simulink model "c"  (R2023a)
settings: Solver=ode4  StartTime=0.0  StopTime=15  FixedStep=0.002  RelTol=1e-3
InitFcn:
  | init;
undefined symbols (not defined in the file): g, N, T, v_c
libraries: dspsrcs4 x2
settings Model: Creator=Ali  LastModifiedBy=Ali

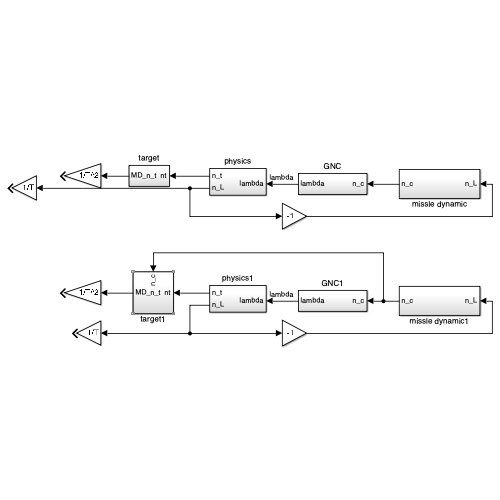
[thumbnail: Simulink's stored preview of the top-level diagram]
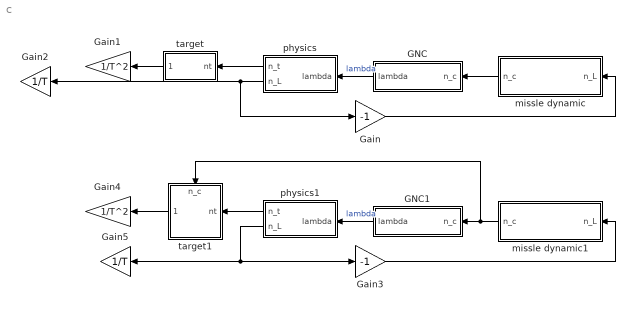
== system c ==
  GNC : Subsystem
  GNC1 : Subsystem
  Gain : Gain  Gain=-1
  Gain1 : Gain  Gain=1/T^2
  Gain2 : Gain  Gain=1/T
  Gain3 : Gain  Gain=-1
  Gain4 : Gain  Gain=1/T^2
  Gain5 : Gain  Gain=1/T
  missle dynamic : Subsystem
  missle dynamic1 : Subsystem
  physics : Subsystem
  physics1 : Subsystem
  target : Subsystem
  target1 : Subsystem
      settings: PortSchema="{\"entries\":[{\"content\":{\"sides\":[{\"content\":{\"connectorIds\":[\"In1\"]},\"type\":\"ConnectorPlacement.EquallySpacedRectSide\",\"uuid\":\"ed75f11e-c865-4004-9925-7377fa04d387\"},{\"content\":{\"connectorIds\":[\"Out1\"],\"side\":\"RIGHT\"},\"type\":\"ConnectorPlacement.EquallySpacedRectSide\",\"uuid\":\"bae2f0f6-1e21-4a13-88c5-2ae7c6156ea9\"},{\"content\":{\"connectorIds\":[\"In2\"],\"side\":\"TOP\"},\"type\":\"ConnectorPlacement.EquallySpacedRectSide\",\"uuid\":\"941d1b82-2a2d-4b33-9910-844af34ed272\"}]},\"type\":\"ConnectorPlacement.EquallySpacedConnector\",\"uuid\":\"c15f6690-1bd4-4323-98c9-9e5b3f44ccd0\"}],\"packageUris\":[\"http://schema.mathworks.com/mf0/Connector/R2020b\"],\"version\":\"1.0\"}"
  wires:
  GNC/1(lambda) -> physics/1(lambda)  "lambda"
  physics/2(n_L) -> Gain2/1, Gain/1
  missle dynamic/1(n_c) -> GNC/1(n_c)
  target/1(MD_n_t) -> Gain1/1
  physics/1(n_t) -> target/1(nt)
  Gain/1 -> missle dynamic/1(n_L)
  target1/1(MD_n_t) -> Gain4/1
  GNC1/1(lambda) -> physics1/1(lambda)  "lambda"
  physics1/1(n_t) -> target1/1(nt)
  physics1/2(n_L) -> Gain5/1, Gain3/1
  missle dynamic1/1(n_c) -> target1/2(n_c), GNC1/1(n_c)
  Gain3/1 -> missle dynamic1/1(n_L)

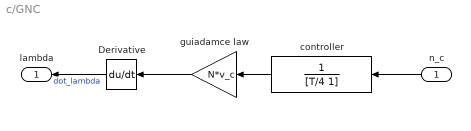
== system c/GNC ==
  n_c : Inport
  Derivative : Derivative
  controller : TransferFcn  Denominator=[T/4 1]
  guiadamce law : Gain  Gain=N*v_c
  lambda : Outport
  wires:
  Derivative/1 -> lambda/1  "dot_lambda"
  n_c/1 -> controller/1
  controller/1 -> guiadamce law/1
  guiadamce law/1 -> Derivative/1

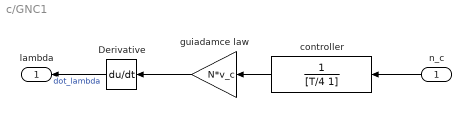
== system c/GNC1 ==
  n_c : Inport
  Derivative : Derivative
  controller : TransferFcn  Denominator=[T/4 1]
  guiadamce law : Gain  Gain=N*v_c
  lambda : Outport
  wires:
  Derivative/1 -> lambda/1  "dot_lambda"
  n_c/1 -> controller/1
  controller/1 -> guiadamce law/1
  guiadamce law/1 -> Derivative/1

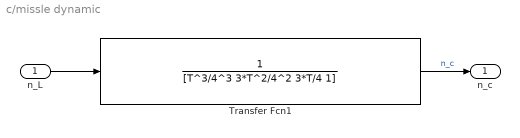
== system c/missle dynamic ==
  n_L : Inport
  Transfer Fcn1 : TransferFcn  Denominator=[T^3/4^3 3*T^2/4^2 3*T/4 1]
  n_c : Outport
  wires:
  Transfer Fcn1/1 -> n_c/1  "n_c"
  n_L/1 -> Transfer Fcn1/1

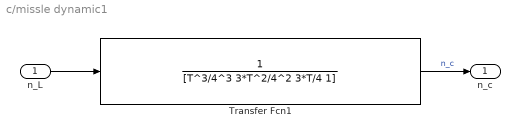
== system c/missle dynamic1 ==
  n_L : Inport
  Transfer Fcn1 : TransferFcn  Denominator=[T^3/4^3 3*T^2/4^2 3*T/4 1]
  n_c : Outport
  wires:
  Transfer Fcn1/1 -> n_c/1  "n_c"
  n_L/1 -> Transfer Fcn1/1

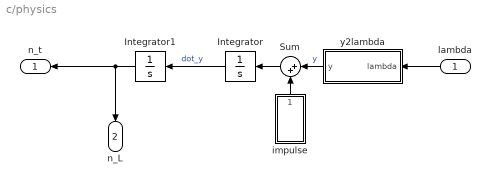
== system c/physics ==
  lambda : Inport
  Integrator : Integrator
  Integrator1 : Integrator
  Sum : Sum  Inputs=|++
  impulse : Subsystem
  y2lambda : Subsystem
  n_t : Outport
  n_L : Outport  Port=2
  wires:
  Integrator/1 -> Integrator1/1  "dot_y"
  Integrator1/1 -> n_L/1, n_t/1
  y2lambda/1(y) -> Sum/1  "y"
  lambda/1 -> y2lambda/1(lambda)
  impulse/1(impulse) -> Sum/2
  Sum/1 -> Integrator/1

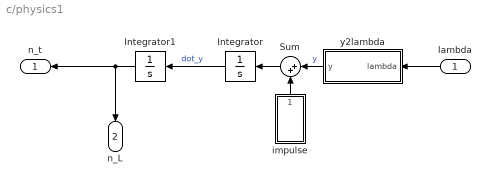
== system c/physics1 ==
  lambda : Inport
  Integrator : Integrator
  Integrator1 : Integrator
  Sum : Sum  Inputs=|++
  impulse : Subsystem
  y2lambda : Subsystem
  n_t : Outport
  n_L : Outport  Port=2
  wires:
  Integrator/1 -> Integrator1/1  "dot_y"
  Integrator1/1 -> n_L/1, n_t/1
  y2lambda/1(y) -> Sum/1  "y"
  lambda/1 -> y2lambda/1(lambda)
  impulse/1(impulse) -> Sum/2
  Sum/1 -> Integrator/1

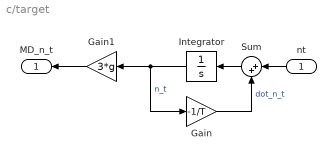
== system c/target ==
  nt : Inport
  Gain : Gain  Gain=-1/T
  Gain1 : Gain  Gain=3*g
  Integrator : Integrator
  Sum : Sum  Inputs=|++
  MD_n_t : Outport
  wires:
  Integrator/1 -> Gain/1, Gain1/1  "n_t"
  Sum/1 -> Integrator/1
  nt/1 -> Sum/1
  Gain/1 -> Sum/2  "dot_n_t"
  Gain1/1 -> MD_n_t/1

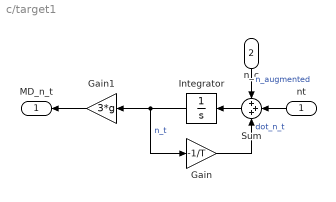
== system c/target1 ==
  nt : Inport
  n_c : Inport  Port=2
  Gain : Gain  Gain=-1/T
  Gain1 : Gain  Gain=3*g
  Integrator : Integrator
  Sum : Sum  Inputs=+++
  MD_n_t : Outport
  wires:
  Integrator/1 -> Gain/1, Gain1/1  "n_t"
  Sum/1 -> Integrator/1
  Gain1/1 -> MD_n_t/1
  Gain/1 -> Sum/3  "dot_n_t"
  nt/1 -> Sum/2
  n_c/1 -> Sum/1  "n_augmented"

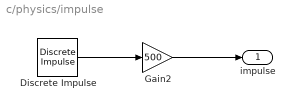
== system c/physics/impulse ==
  Discrete Impulse : dspsrcs4/Discrete  Impulse  Delay=0  SampleTime=0.002  FrameSample=1  OutputFrames=off  dataType=double  isSigned=on  wordLen=16  udDataType=sfix(16)  fracBitsMode=Best precision  numFracBits=15  OutDataTypeStr=double  LastOutDataTypeStr=double
  Gain2 : Gain  Gain=500
  impulse : Outport
  wires:
  Gain2/1 -> impulse/1
  Discrete Impulse/1 -> Gain2/1

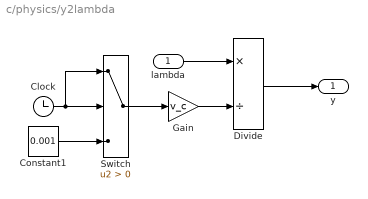
== system c/physics/y2lambda ==
  lambda : Inport
  Clock : Clock
  Constant1 : Constant  Value=0.001
  Divide : Product  Inputs=*/
  Gain : Gain  Gain=v_c
  Switch : Switch  Criteria=u2 > Threshold  SaturateOnIntegerOverflow=off  InputSameDT=off
  y : Outport
  wires:
  Gain/1 -> Divide/2
  lambda/1 -> Divide/1
  Divide/1 -> y/1
  Constant1/1 -> Switch/3
  Clock/1 -> Switch/1, Switch/2
  Switch/1 -> Gain/1

== system c/physics1/impulse ==
  Discrete Impulse : dspsrcs4/Discrete  Impulse  Delay=0  SampleTime=0.002  FrameSample=1  OutputFrames=off  dataType=double  isSigned=on  wordLen=16  udDataType=sfix(16)  fracBitsMode=Best precision  numFracBits=15  OutDataTypeStr=double  LastOutDataTypeStr=double
  Gain2 : Gain  Gain=500
  impulse : Outport
  wires:
  Gain2/1 -> impulse/1
  Discrete Impulse/1 -> Gain2/1

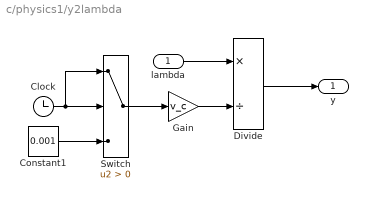
== system c/physics1/y2lambda ==
  lambda : Inport
  Clock : Clock
  Constant1 : Constant  Value=0.001
  Divide : Product  Inputs=*/
  Gain : Gain  Gain=v_c
  Switch : Switch  Criteria=u2 > Threshold  SaturateOnIntegerOverflow=off  InputSameDT=off
  y : Outport
  wires:
  Gain/1 -> Divide/2
  lambda/1 -> Divide/1
  Divide/1 -> y/1
  Constant1/1 -> Switch/3
  Clock/1 -> Switch/1, Switch/2
  Switch/1 -> Gain/1
